simulink model "FurutaSimulink2"  (R2017a)
settings: Solver=ode5  StartTime=0.0  StopTime=40  FixedStep=dtSim  RelTol=1e-3
values from neighbouring files (symbols this model uses):
  a = SVMModel.Alpha    [SVM.m]
  alpha = J + (M + 1/3*ma+mp)*la^2    (= 0.0100418552736)    [FurutaConstants.m]    (also in FurutaConstantsSymb.m = 0.109041855274; FurutaSymb2.m = 0.109041855274; myStateTransitionFcn.m = 0.0103073912861)
  b2 = 5.52e-04    (= 0.000552)    [FurutaConstants.m]    (also in FurutaConstantsSymb.m; FurutaSymb2.m; myStateTransitionFcn.m)
  beta = (M + 1/3*mp)*lp^2    (= 0.000947879666364)    [FurutaConstants.m]    (also in FurutaConstantsSymb.m; FurutaSymb2.m; myStateTransitionFcn.m = 0.00123523203086)
  delta = (M + .5*mp)*g*lp    (= 0.058182327162)    [FurutaConstants.m]    (also in FurutaConstantsSymb.m; FurutaSymb2.m; myStateTransitionFcn.m = 0.069941083662)
  dtDisc = 0.05    [FurutaConstants.m]    (also in FurutaSymb2.m = 0.01)
  g = 9.81    [FurutaConstants.m]    (also in FurutaConstantsSymb.m; FurutaSymb2.m; myStateTransitionFcn.m)
  gamma = (M + .5*mp)*la*lp    (= 0.00136678056009)    [FurutaConstants.m]    (also in FurutaConstantsSymb.m; FurutaSymb2.m; myStateTransitionFcn.m = 0.00164300945259)
  J = 0.001    [FurutaConstants.m]    (also in FurutaConstantsSymb.m = 0.1; FurutaSymb2.m = 0.1; myStateTransitionFcn.m)
  K = 0.182    [FurutaConstants.m]    (also in FurutaConstantsSymb.m = place(A,B,p); FurutaSymb2.m = 0.01; myStateTransitionFcn.m)
  Kc = place(A,B,[-2+2i -2-2i -1 -4])    [FurutaConstants.m]
  la = 230.45e-3    (= 0.23045)    [FurutaConstants.m]    (also in FurutaConstantsSymb.m; FurutaSymb2.m; Visualisation.m; myStateTransitionFcn.m)
  lp = 239.73e-3    (= 0.23973)    [FurutaConstants.m]    (also in FurutaConstantsSymb.m; FurutaSymb2.m; myStateTransitionFcn.m)
  M = 0    [FurutaConstants.m]    (also in FurutaConstantsSymb.m; FurutaSymb2.m; Visualisation2.m = scatter3(Xv(2),Yv(2),Zv(2),s,'filled','MarkerFaceColor','b',; Visualisation3.m = scatter3(Xv(2),Yv(2),Zv(2),s,'filled','MarkerFaceColor','b',)
  ma = 0.36233    [FurutaConstants.m]    (also in FurutaConstantsSymb.m; FurutaSymb2.m; myStateTransitionFcn.m)
  mp = 0.04948    [FurutaConstants.m]    (also in FurutaConstantsSymb.m; FurutaSymb2.m; myStateTransitionFcn.m)
  PotMax = .5*mp*lp*g    (= 0.058182327162)    [FurutaConstants.m]
  R = 12.38    [FurutaConstants.m]    (also in FurutaConstantsSymb.m; FurutaSymb2.m; myStateTransitionFcn.m)
  sigma = SVMModel.KernelParameters.Scale    [SVM.m]
  Thetao = angle*pi/180    (= 0.261799387799)    [FurutaConstants.m]
  xs = SVMModel.SupportVectors    [SVM.m]
  xt = [theta2o, dtheta1o, dtheta2o]    [SVM.m]
  ys = SVMModel.SupportVectorLabels    [SVM.m]
undefined symbols (not defined in the file or in its folder): A3, Aaa, Aab, Aba, Abb, B3, Ba, Bb, C3, Kc2, Ke, L, xs1, xs2, xs3
settings Model: Creator=NSEE  LastModifiedBy=felip
settings DataIOCC: LimitDataPoints=on  SaveFormat=Array
settings OptimizationCC: LifeSpan=inf
settings DebuggingCC: SFUnexpectedBacktrackingDiag=warning  SFNoUnconditionalDefaultTransitionDiag=warning  SFExecutionAtInitializationDiag=none
settings HardwareCC: ProdBitPerPointer=32  ProdBitPerSizeT=32  ProdBitPerPtrDiffT=32  ProdLargestAtomicFloat=None  ProdIntDivRoundTo=Undefined  ProdEndianess=Unspecified  ProdWordSize=32  ProdHWDeviceType=32-bit Generic
settings ModelReferenceCC: PropagateSignalLabelsOutOfModel=off
settings GRTTargetCC: TargetLangStandard=C89/C90 (ANSI)  GeneratePreprocessorConditionals=Disable all
settings ConfigComp: CovMetricSettings=dw  CovHtmlReporting=on  CovSaveCumulativeToWorkspaceVar=on  CovSaveSingleToWorkspaceVar=on  CovExternalEMLEnable=off

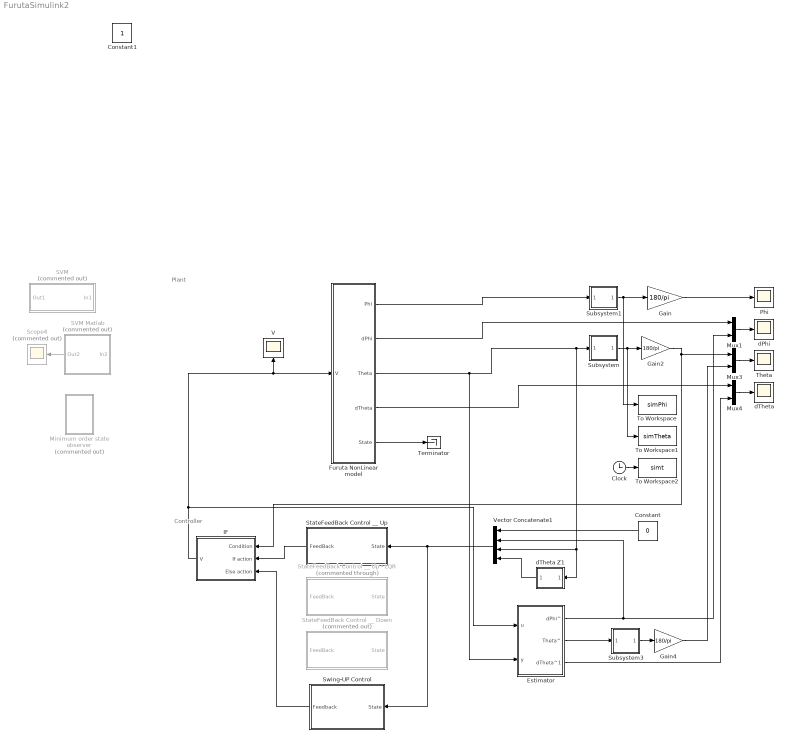
== system FurutaSimulink2 ==
  note: Plant
  note: Controller
  Clock : Clock
  Constant : Constant  Value=0
  Estimator : Subsystem
  Furuta NonLinear model : Subsystem
  Gain : Gain  Gain=180/pi
  Gain2 : Gain  Gain=180/pi
  Gain4 : Gain  Gain=180/pi
  IF : Subsystem
  "Minimum order state observer " : Subsystem  Commented=on
  Mux1 : Mux  Inputs=2
  Mux3 : Mux  Inputs=2
  Mux4 : Mux  Inputs=2
  Phi : Scope
  SVM : Subsystem  Commented=on  TreatAsAtomicUnit=on
  SVM Matlab : Subsystem  Commented=on
  Scope4 : Scope  Commented=on
  StateFeedBack Control __ Down : Subsystem  Commented=on
  StateFeedBack Control __ Up : Subsystem
  StateFeedBack Control __ Up - LQR : Subsystem  Commented=through
  Subsystem : Subsystem
  Subsystem1 : Subsystem
  Subsystem3 : Subsystem
  Swing-UP Control : Subsystem
  Terminator : Terminator
  Theta : Scope
  To Workspace : ToWorkspace  VariableName=simPhi  SampleTime=-1
      settings: Save2DSignal=2-D array (concatenate along first dimension)
  To Workspace1 : ToWorkspace  VariableName=simTheta  SampleTime=-1
      settings: Save2DSignal=2-D array (concatenate along first dimension)
  To Workspace2 : ToWorkspace  VariableName=simt  SampleTime=-1
      settings: Save2DSignal=2-D array (concatenate along first dimension)
  V : Scope
  Vector Concatenate1 : Concatenate  NumInputs=4
  dPhi : Scope
  dTheta : Scope
  dTheta Z1 : Subsystem
  Constant1 : Constant  IOType=siggen
  wires:
  Furuta NonLinear model/1("Phi ") -> Subsystem1/1(In1)
  SVM Matlab/1(Out2) -> Scope4/1
  Subsystem/1(Out1) -> To Workspace1/1, Gain2/1
  Subsystem1/1(Out1) -> To Workspace/1, Gain/1
  Gain2/1 -> Mux3/1, IF/1(Condition)
  StateFeedBack Control __ Up/1(FeedBack) -> IF/2("If action ")
  IF/1(V) -> V/1, Furuta NonLinear model/1(V), Estimator/1(u)
  Clock/1 -> To Workspace2/1
  Mux1/1 -> dPhi/1
  Furuta NonLinear model/2("dPhi ") -> Mux1/1
  Mux3/1 -> Theta/1
  Mux4/1 -> dTheta/1
  Furuta NonLinear model/4("dTheta ") -> Mux4/1
  Swing-UP Control/1(Feedback) -> IF/3(Else action)
  Gain/1 -> Phi/1
  Gain4/1 -> Mux3/2
  Furuta NonLinear model/3("Theta ") -> Estimator/2(y), Vector Concatenate1/3, dTheta Z1/1(In1), Subsystem/1(In1)
  Constant/1 -> Vector Concatenate1/1
  Vector Concatenate1/1 -> Swing-UP Control/1(State), StateFeedBack Control __ Up/1(State)
  dTheta Z1/1(Out1) -> Vector Concatenate1/4
  Subsystem3/1(Out1) -> Gain4/1
  Estimator/1(dPhi^) -> Mux1/2, Vector Concatenate1/2
  Estimator/2(Theta^) -> Subsystem3/1(In1)
  Estimator/3(dTheta^1) -> Mux4/2
  Furuta NonLinear model/5(State) -> Terminator/1

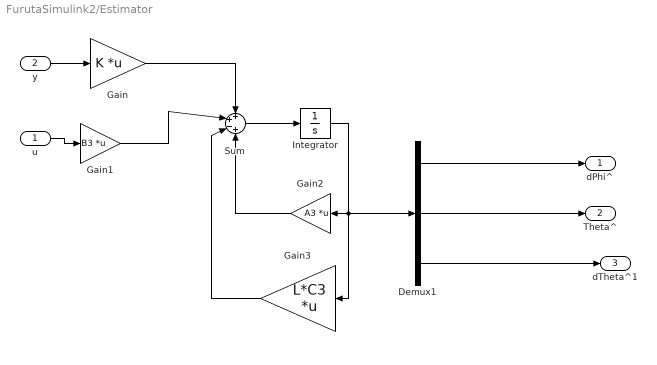
== system FurutaSimulink2/Estimator ==
  u : Inport
  y : Inport  Port=2
  Demux1 : Demux  Outputs=3
  Gain : Gain  Gain=K  Multiplication=Matrix(K*u)
  Gain1 : Gain  Gain=B3  Multiplication=Matrix(K*u)
  Gain2 : Gain  Gain=A3  Multiplication=Matrix(K*u)
  Gain3 : Gain  Gain=L*C3  Multiplication=Matrix(K*u)
  Integrator : Integrator
  Sum : Sum  Inputs=++-+
  dPhi^ : Outport
  Theta^ : Outport  Port=2
  dTheta^1 : Outport  Port=3
  wires:
  y/1 -> Gain/1
  Gain/1 -> Sum/1
  u/1 -> Gain1/1
  Gain1/1 -> Sum/2
  Sum/1 -> Integrator/1
  Gain2/1 -> Sum/4
  Gain3/1 -> Sum/3
  Integrator/1 -> Demux1/1, Gain3/1, Gain2/1
  Demux1/1 -> dPhi^/1
  Demux1/3 -> dTheta^1/1
  Demux1/2 -> Theta^/1

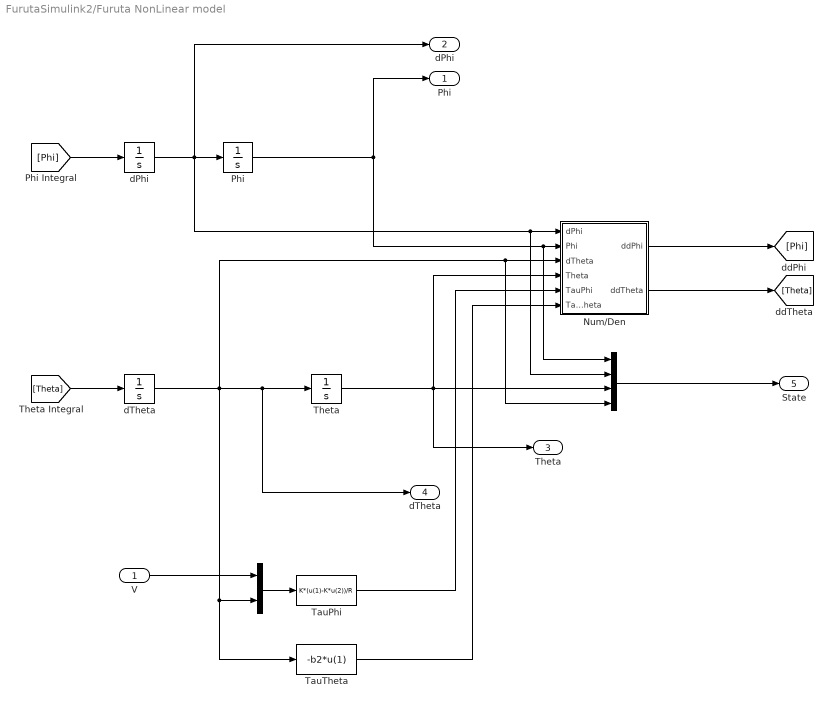
== system FurutaSimulink2/Furuta NonLinear model ==
  V : Inport
  " " : Concatenate
  " " : Concatenate  NumInputs=4
  Num/Den : Subsystem
  Phi : Integrator
  TauPhi : Fcn  Expr=K*(u(1)-K*u(2))/R
  TauTheta : Fcn  Expr=-b2*u(1)
  Theta : Integrator  InitialCondition=Thetao  WrappedStateUpperValue=2*pi  WrappedStateLowerValue=0
  dPhi : Integrator
  dTheta : Integrator
  "Phi " : Outport
  "dPhi " : Outport  Port=2
  "Theta " : Outport  Port=3
  "dTheta " : Outport  Port=4
  State : Outport  Port=5
  wires:
  dTheta/1 -> Theta/1, "dTheta "/1, " "/4, Num/Den/3(dTheta), TauTheta/1, " "/2
  [Theta] -> dTheta/1
  dPhi/1 -> Phi/1, "dPhi "/1, " "/2, Num/Den/1(dPhi)
  [Phi] -> dPhi/1
  TauPhi/1 -> Num/Den/5(TauPhi)
  V/1 -> " "/1
  TauTheta/1 -> Num/Den/6(TauTheta)
  " "/1 -> TauPhi/1
  " "/1 -> State/1
  Num/Den/1(ddPhi) -> [Phi]
  Num/Den/2(ddTheta) -> [Theta]
  Theta/1 -> Num/Den/4("Theta "), "Theta "/1, " "/3
  Phi/1 -> " "/1, Num/Den/2(Phi), "Phi "/1

== system FurutaSimulink2/IF ==
  Condition : Inport
  "If action " : Inport  Port=2
  Else action : Inport  Port=3
  If : If  IfExpression=(u1 < 210) & (u1 > 150)
  If Action Subsystem : Subsystem  TreatAsAtomicUnit=on
  If Action Subsystem1 : Subsystem  TreatAsAtomicUnit=on
  Merge : Merge
  V : Outport
  wires:
  If/2 -> If Action Subsystem1/Action
  If/1 -> If Action Subsystem/Action
  "If action "/1 -> If Action Subsystem/1(In1)
  If Action Subsystem1/1(Out1) -> Merge/2
  Else action/1 -> If Action Subsystem1/1(In1)
  Merge/1 -> V/1
  If Action Subsystem/1(Out1) -> Merge/1
  Condition/1 -> If/1

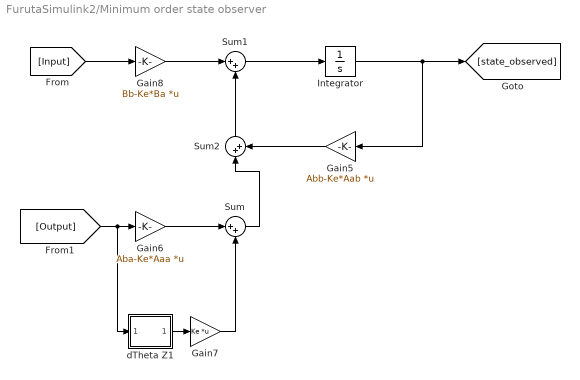
== system FurutaSimulink2/Minimum order state observer  ==
  Gain5 : Gain  Gain=Abb-Ke*Aab  Multiplication=Matrix(K*u)
  Gain6 : Gain  Gain=Aba-Ke*Aaa  Multiplication=Matrix(K*u)
  Gain7 : Gain  Gain=Ke  Multiplication=Matrix(K*u)
  Gain8 : Gain  Gain=Bb-Ke*Ba  Multiplication=Matrix(K*u)
  Integrator : Integrator
  Sum : Sum  Inputs=|++
  Sum1 : Sum  Inputs=|++
  Sum2 : Sum  Inputs=|++
  dTheta Z1 : Subsystem
  wires:
  [Input] -> Gain8/1
  Integrator/1 -> [state_observed], Gain5/1
  Gain5/1 -> Sum2/2
  Sum1/1 -> Integrator/1
  Gain7/1 -> Sum/2
  Gain6/1 -> Sum/1
  [Output] -> dTheta Z1/1(In1), Gain6/1
  Gain8/1 -> Sum1/1
  Sum/1 -> Sum2/1
  Sum2/1 -> Sum1/2
  dTheta Z1/1(Out1) -> Gain7/1

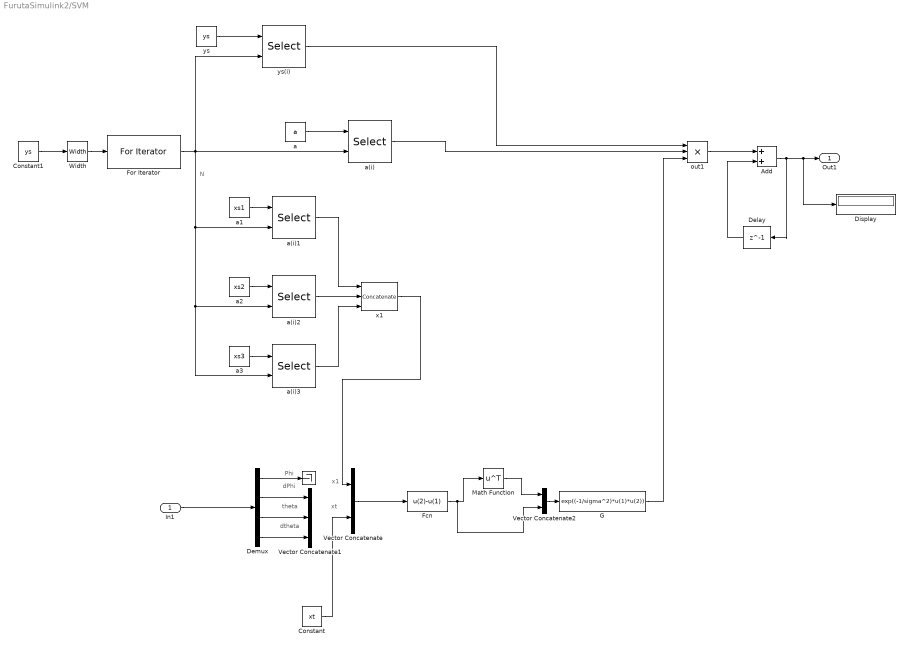
== system FurutaSimulink2/SVM ==
  note: x1
  note: xt
  note: N
  note: Phi
  note: dtheta
  note: theta
  note: dPhi
  In1 : Inport
  " " : Terminator
  Add : Sum
  Constant : Constant  Value=xt
  Constant1 : Constant  Value=ys
  Delay : Delay  DelayLength=1  InitialCondition=0
  Demux : Demux
  Display : Display
  Fcn : Fcn  Expr=u(2)-u(1)
  For Iterator : ForIterator  IterationSource=external  IndexMode=Zero-based
  G : Fcn  Expr=exp((-1/sigma^2)*u(1)*u(2))
  Math Function : Math  Operator=transpose  SaturateOnIntegerOverflow=on
  Vector Concatenate : Concatenate
  Vector Concatenate1 : Concatenate  NumInputs=3
  Vector Concatenate2 : Concatenate
  Width : Width
  a : Constant  Value=a
  a(i){,1..3} (4 alike) : Selector  IndexMode=Zero-based  InputPortWidth=2152  IndexOptions=Index vector (port)  Indices=[1 3]  OutputSizes=1
  a1 : Constant  Value=xs1
  a2 : Constant  Value=xs2
  a3 : Constant  Value=xs3
  out1 : Product  Inputs=3
  x1 : Concatenate  NumInputs=3  ConcatenateDimension=2
  ys : Constant  Value=ys
  ys(i) : Selector  IndexMode=Zero-based  InputPortWidth=2152  IndexOptions=Index vector (port)  Indices=[1 3]  OutputSizes=1
  Out1 : Outport
  wires:
  Width/1 -> For Iterator/1
  Constant1/1 -> Width/1
  In1/1 -> Demux/1
  Demux/1 -> " "/1
  Demux/2 -> Vector Concatenate1/1
  Demux/3 -> Vector Concatenate1/2
  Demux/4 -> Vector Concatenate1/3
  ys(i)/1 -> out1/1
  out1/1 -> Add/1
  Add/1 -> Display/1, Out1/1, Delay/1
  Fcn/1 -> Math Function/1, Vector Concatenate2/2
  Vector Concatenate/1 -> Fcn/1
  Math Function/1 -> Vector Concatenate2/1
  Vector Concatenate2/1 -> G/1
  G/1 -> out1/3
  ys/1 -> ys(i)/1
  a/1 -> a(i)/1
  a(i)/1 -> out1/2
  a1/1 -> a(i)1/1
  a2/1 -> a(i)2/1
  For Iterator/1 -> a(i)2/2, a(i)3/2, a(i)1/2, a(i)/2, ys(i)/2
  a3/1 -> a(i)3/1
  a(i)2/1 -> x1/2
  a(i)1/1 -> x1/1
  a(i)3/1 -> x1/3
  x1/1 -> Vector Concatenate/1
  Constant/1 -> Vector Concatenate/2
  Delay/1 -> Add/2

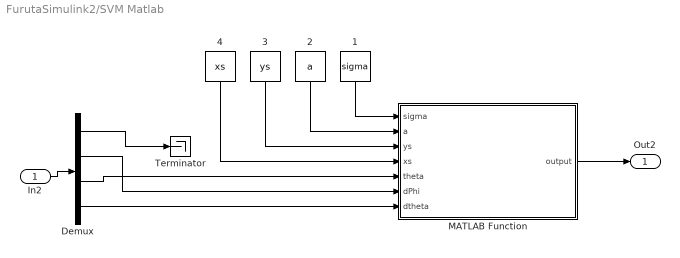
== system FurutaSimulink2/SVM Matlab ==
  In2 : Inport
  1 : Constant  Value=sigma
  2 : Constant  Value=a
  3 : Constant  Value=ys
  4 : Constant  Value=xs
  Demux : Demux
  MATLAB Function : MATLAB Function  TreatAsAtomicUnit=on
  Terminator : Terminator
  Out2 : Outport
  wires:
  3/1 -> MATLAB Function/3(ys)
  1/1 -> MATLAB Function/1(sigma)
  2/1 -> MATLAB Function/2(a)
  4/1 -> MATLAB Function/4(xs)
  In2/1 -> Demux/1
  MATLAB Function/1(output) -> Out2/1
  Demux/1 -> Terminator/1
  Demux/2 -> MATLAB Function/6(dPhi)
  Demux/3 -> MATLAB Function/5(theta)
  Demux/4 -> MATLAB Function/7(dtheta)

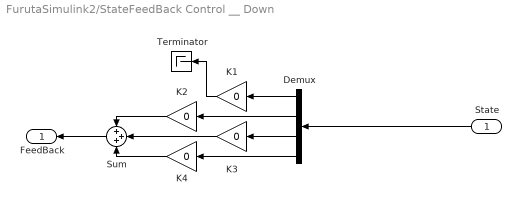
== system FurutaSimulink2/StateFeedBack Control __ Down ==
  State : Inport
  Demux : Demux
  K{1..4} (4 alike) : Gain  Gain=0
  Sum : Sum  Inputs=+++
  Terminator : Terminator
  FeedBack : Outport
  wires:
  K2/1 -> Sum/1
  Demux/3 -> K3/1
  Sum/1 -> FeedBack/1
  State/1 -> Demux/1
  K3/1 -> Sum/2
  Demux/1 -> K1/1
  Demux/2 -> K2/1
  Demux/4 -> K4/1
  K4/1 -> Sum/3
  K1/1 -> Terminator/1

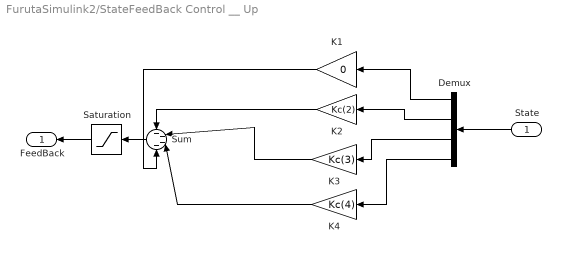
== system FurutaSimulink2/StateFeedBack Control __ Up ==
  State : Inport
  Demux : Demux
  K1 : Gain  Gain=0
  K2 : Gain  Gain=Kc(2)
  K3 : Gain  Gain=Kc(3)
  K4 : Gain  Gain=Kc(4)
  Saturation : Saturate  UpperLimit=12  LowerLimit=-12
  Sum : Sum  Inputs=----
  FeedBack : Outport
  wires:
  K2/1 -> Sum/1
  Demux/3 -> K3/1
  Sum/1 -> Saturation/1
  State/1 -> Demux/1
  K3/1 -> Sum/2
  Demux/1 -> K1/1
  Demux/2 -> K2/1
  Demux/4 -> K4/1
  K4/1 -> Sum/3
  Saturation/1 -> FeedBack/1
  K1/1 -> Sum/4

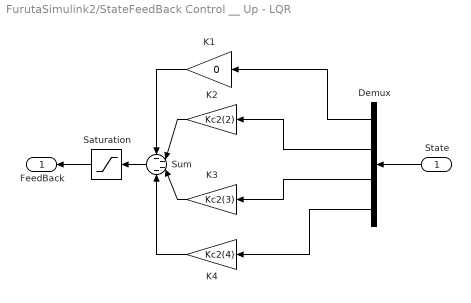
== system FurutaSimulink2/StateFeedBack Control __ Up - LQR ==
  State : Inport
  Demux : Demux
  K1 : Gain  Gain=0
  K2 : Gain  Gain=Kc2(2)
  K3 : Gain  Gain=Kc2(3)
  K4 : Gain  Gain=Kc2(4)
  Saturation : Saturate  UpperLimit=12  LowerLimit=-12
  Sum : Sum  Inputs=----
  FeedBack : Outport
  wires:
  Sum/1 -> Saturation/1
  State/1 -> Demux/1
  Demux/4 -> K4/1
  Saturation/1 -> FeedBack/1
  K1/1 -> Sum/1
  K4/1 -> Sum/4
  K3/1 -> Sum/3
  K2/1 -> Sum/2
  Demux/1 -> K1/1
  Demux/2 -> K2/1
  Demux/3 -> K3/1

== system FurutaSimulink2/Subsystem ==
  In1 : Inport
  2pi : Constant  Value=2*pi
  Add : Sum
  Constant : Constant  Value=-pi
  Math Function : Math  Operator=mod  SaturateOnIntegerOverflow=on
  Out1 : Outport
  wires:
  Math Function/1 -> Out1/1
  2pi/1 -> Math Function/2
  Constant/1 -> Add/2
  In1/1 -> Add/1
  Add/1 -> Math Function/1

== system FurutaSimulink2/Subsystem1 ==
  In1 : Inport
  2pi : Constant  Value=2*pi
  Math Function : Math  Operator=mod  SaturateOnIntegerOverflow=on
  Out1 : Outport
  wires:
  2pi/1 -> Math Function/2
  Math Function/1 -> Out1/1
  In1/1 -> Math Function/1

== system FurutaSimulink2/Subsystem3 ==
  In1 : Inport
  2pi : Constant  Value=2*pi
  Add : Sum
  Constant : Constant  Value=-pi
  Math Function : Math  Operator=mod  SaturateOnIntegerOverflow=on
  Out1 : Outport
  wires:
  Math Function/1 -> Out1/1
  2pi/1 -> Math Function/2
  Constant/1 -> Add/2
  In1/1 -> Add/1
  Add/1 -> Math Function/1

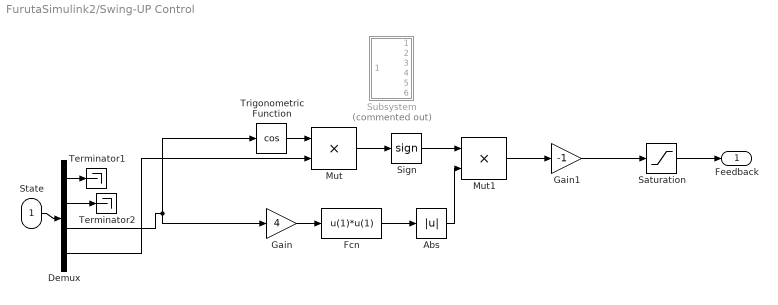
== system FurutaSimulink2/Swing-UP Control ==
  State : Inport
  Abs : Abs
  Demux : Demux
  Fcn : Fcn  Expr=u(1)*u(1)
  Gain : Gain  Gain=4
  Gain1 : Gain  Gain=-1
  Mut : Product  Inputs=**
  Mut1 : Product  Inputs=**
  Saturation : Saturate  UpperLimit=12  LowerLimit=-12
  Sign : Signum
  Subsystem : Subsystem  Commented=on
  Terminator1 : Terminator
  Terminator2 : Terminator
  Trigonometric Function : Trigonometry  Operator=cos
  Feedback : Outport
  wires:
  Saturation/1 -> Feedback/1
  State/1 -> Demux/1
  Gain/1 -> Fcn/1
  Mut/1 -> Sign/1
  Sign/1 -> Mut1/1
  Abs/1 -> Mut1/2
  Demux/4 -> Mut/2
  Trigonometric Function/1 -> Mut/1
  Fcn/1 -> Abs/1
  Demux/3 -> Gain/1, Trigonometric Function/1
  Mut1/1 -> Gain1/1
  Gain1/1 -> Saturation/1
  Demux/1 -> Terminator1/1
  Demux/2 -> Terminator2/1

== system FurutaSimulink2/dTheta Z1 ==
  In1 : Inport
  Delay : Delay  InitialCondition=0  SampleTime=dtDisc
  Delay1 : Delay  DelayLength=1  InitialCondition=0  SampleTime=dtDisc
  Delay3 : Delay  DelayLength=0  InitialCondition=0  SampleTime=dtDisc
  Fcn1 : Fcn  Expr=(-u(3)+4*(u(2))-3*(u(1)))/dtDisc
  Gain1 : Gain  Gain=1/2
  Vector Concatenate : Concatenate  NumInputs=3
  Out1 : Outport
  wires:
  Fcn1/1 -> Gain1/1
  Delay1/1 -> Vector Concatenate/2
  Vector Concatenate/1 -> Fcn1/1
  Delay/1 -> Vector Concatenate/1
  Delay3/1 -> Vector Concatenate/3
  Gain1/1 -> Out1/1
  In1/1 -> Delay1/1, Delay/1, Delay3/1

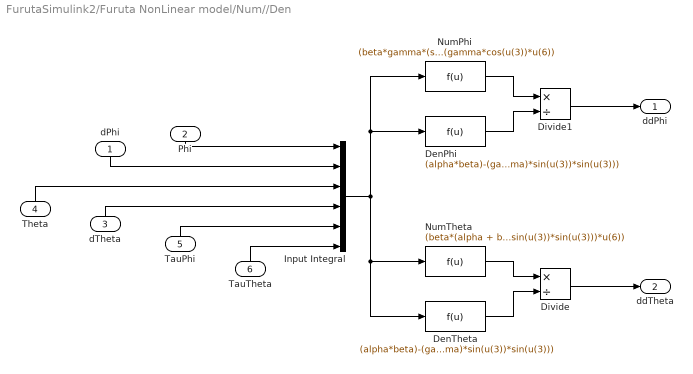
== system FurutaSimulink2/Furuta NonLinear model/Num//Den ==
  dPhi : Inport
  Phi : Inport  Port=2
  dTheta : Inport  Port=3
  "Theta " : Inport  Port=4
  TauPhi : Inport  Port=5
  TauTheta : Inport  Port=6
  DenPhi : Fcn  Expr=(alpha*beta)-(gamma*gamma)+((beta*beta+gamma*gamma)*sin(u(3))*sin(u(3)))
  DenTheta : Fcn  Expr=(alpha*beta)-(gamma*gamma)+((beta*beta+gamma*gamma)*sin(u(3))*sin(u(3)))
  Divide : Product  Inputs=*/
  Divide1 : Product  Inputs=*/
  Input Integral : Concatenate  NumInputs=6
  NumPhi : Fcn  Expr=(beta*gamma*(sin(u(3))*sin(u(3))-1)*cos(u(3))*sin(u(3))*u(2)*u(2)) - (2*beta*beta*cos(u(3))*sin(u(3))*u(2)*u(4)) + ( beta*gamma*sin(u(3))*u(4)*u(4)) - (gamma*delta*cos(u(3))*sin(u(3))) + (beta*u(5)) - (gamma*cos(u(3))*u(6))
  NumTheta : Fcn  Expr=(beta*(alpha + beta*sin(u(3))*sin(u(3)))*cos(u(3))*sin(u(3))*u(2)*u(2))+(2*beta*gamma*(1-sin(u(3))*sin(u(3)))*sin(u(3))*u(2)*u(4))-( gamma*gamma*cos(u(3))*sin(u(3))*u(4)*u(4))+( delta*(alpha+beta*sin(u(3))*sin(u(3)))*sin(u(3)))-(gamma*cos(u(3))*u(5))+((alpha+beta*sin(u(3))*sin(u(3)))*u(6))
  ddPhi : Outport
  ddTheta : Outport  Port=2
  wires:
  NumTheta/1 -> Divide/1
  DenTheta/1 -> Divide/2
  DenPhi/1 -> Divide1/2
  NumPhi/1 -> Divide1/1
  Divide1/1 -> ddPhi/1
  Divide/1 -> ddTheta/1
  dPhi/1 -> Input Integral/2
  Phi/1 -> Input Integral/1
  TauTheta/1 -> Input Integral/6
  dTheta/1 -> Input Integral/4
  TauPhi/1 -> Input Integral/5
  "Theta "/1 -> Input Integral/3
  Input Integral/1 -> NumPhi/1, DenPhi/1, NumTheta/1, DenTheta/1

== system FurutaSimulink2/IF/If Action Subsystem ==
  In1 : Inport
  Action Port : ActionPort  ActionType=then
  Out1 : Outport
  wires:
  In1/1 -> Out1/1

== system FurutaSimulink2/IF/If Action Subsystem1 ==
  In1 : Inport
  Action Port : ActionPort  ActionType=else
  Out1 : Outport  InitialOutput=0
  wires:
  In1/1 -> Out1/1

== system FurutaSimulink2/Minimum order state observer /dTheta Z1 ==
  In1 : Inport
  Delay : Delay  InitialCondition=0  SampleTime=dtDisc
  Delay1 : Delay  DelayLength=1  InitialCondition=0  SampleTime=dtDisc
  Delay3 : Delay  DelayLength=0  InitialCondition=0  SampleTime=dtDisc
  Fcn1 : Fcn  Expr=(-u(3)+4*(u(2))-3*(u(1)))/dtDisc
  Gain1 : Gain  Gain=1/2
  Vector Concatenate : Concatenate  NumInputs=3
  Out1 : Outport
  wires:
  Fcn1/1 -> Gain1/1
  Delay1/1 -> Vector Concatenate/2
  Vector Concatenate/1 -> Fcn1/1
  Delay/1 -> Vector Concatenate/1
  Delay3/1 -> Vector Concatenate/3
  Gain1/1 -> Out1/1
  In1/1 -> Delay1/1, Delay/1, Delay3/1

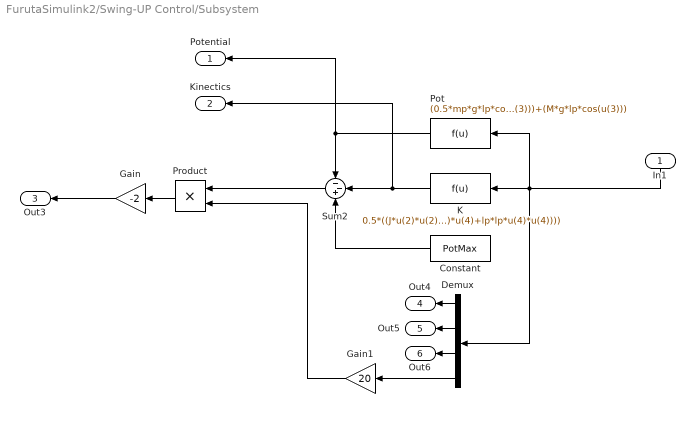
== system FurutaSimulink2/Swing-UP Control/Subsystem ==
  In1 : Inport
  Constant : Constant  Value=PotMax
  Demux : Demux
  Gain : Gain  Gain=-2
  Gain1 : Gain  Gain=20
  K : Fcn  Expr=0.5*((J*u(2)*u(2))+(ma*la*la*u(2)*u(2)/3)+(mp*(la*la+lp*lp*sin(u(3))*sin(u(3))/3)*u(2)*u(2))+(mp*la*lp*cos(u(3))*u(2)*u(4))+(mp*lp*lp*u(4)*u(4)/3)+(M*((la*la+lp*lp*sin(u(3))*sin(u(3)))*u(2)*u(2)+2*la*lp*cos(u(3))*u(2)*u(4)+lp*lp*u(4)*u(4))))
  Pot : Fcn  Expr=(0.5*mp*g*lp*cos(u(3)))+(M*g*lp*cos(u(3)))
  Product : Product
  Sum2 : Sum  Inputs=--+
  Potential : Outport
  Kinectics : Outport  Port=2
  Out3 : Outport  Port=3
  Out4 : Outport  Port=4
  Out5 : Outport  Port=5
  Out6 : Outport  Port=6
  wires:
  Demux/3 -> Out6/1
  Demux/2 -> Out5/1
  Demux/1 -> Out4/1
  Pot/1 -> Potential/1, Sum2/1
  Constant/1 -> Sum2/3
  K/1 -> Kinectics/1, Sum2/2
  Gain/1 -> Out3/1
  Gain1/1 -> Product/2
  In1/1 -> Demux/1, Pot/1, K/1
  Sum2/1 -> Product/1
  Demux/4 -> Gain1/1
  Product/1 -> Gain/1

== matlab function FurutaSimulink2/SVM Matlab/MATLAB Function ==
  data: sigma input; a input; ys input; xs input; output output; theta input; dPhi input; dtheta input
function output = SVM_calculate(sigma,a,ys,xs,theta,dPhi,dtheta)

xt = [theta, dPhi, dtheta];

out = 0;

for i = 1 : length(ys)
    x1 = xs(i,:);
    G = exp((-1/sigma^2)*(xt-x1)*(xt-x1)');
    out1 = a(i)*ys(i)*G;
    out = out + out1;
end

output = out*1000
